simulink model "IF_with_EnabledSS"  (Simulink 9.0)
settings: Solver=FixedStepDiscrete  StartTime=0.0  StopTime=1  FixedStep=0.020000  MaxStep=1  RelTol=1e-3  EnableMultiTasking=on
model workspace (MAT data in the model file):
  x : num (value not decoded)
settings Model: SuppressorTable=22 serialization::archive 11 0 6 0 0 0 0 0  Creator=arnaud  LastModifiedBy=hbourbou
settings DataIOCC: LimitDataPoints=on  SaveFormat=Structure
settings DebuggingCC: UnderspecifiedInitializationDetection=Simplified  MergeDetectMultiDrivingBlocksExec=error  SolverPrmCheckMsg=warning
settings GRTTargetCC: GeneratePreprocessorConditionals=Disable all
settings ConfigComp: CovSFcnEnable=off

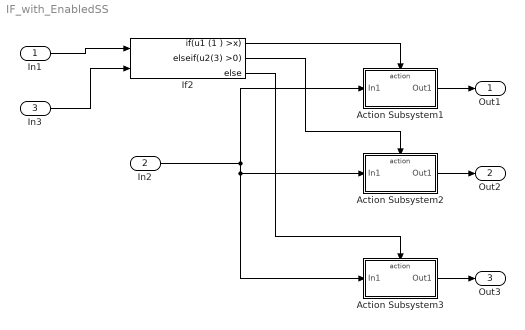
== system IF_with_EnabledSS ==
  In1 : Inport  PortDimensions=3
  In2 : Inport  Port=2
  In3 : Inport  Port=3  OutDataTypeStr=int32  PortDimensions=3
  Action Subsystem1 : Subsystem  TreatAsAtomicUnit=on
  Action Subsystem2 : Subsystem  TreatAsAtomicUnit=on
  Action Subsystem3 : Subsystem  TreatAsAtomicUnit=on
  If2 : If  NumInputs=2  IfExpression=u1 (1 ) >x  ElseIfExpressions=u2(3) >0
  Out1 : Outport
  Out2 : Outport  Port=2
  Out3 : Outport  Port=3
  wires:
  If2/1 -> Action Subsystem1/Action
  In1/1 -> If2/1
  If2/2 -> Action Subsystem2/Action
  Action Subsystem1/1(Out1) -> Out1/1
  Action Subsystem2/1(Out1) -> Out2/1
  In2/1 -> Action Subsystem3/1(In1), Action Subsystem2/1(In1), Action Subsystem1/1(In1)
  In3/1 -> If2/2
  If2/3 -> Action Subsystem3/Action
  Action Subsystem3/1(Out1) -> Out3/1

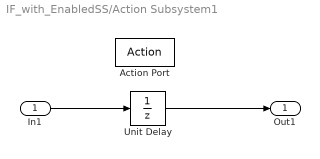
== system IF_with_EnabledSS/Action Subsystem1 ==
  In1 : Inport
  Action Port : ActionPort  InitializeStates=reset  ActionType=then
  Unit Delay : UnitDelay  SampleTime=-1
  Out1 : Outport
  wires:
  In1/1 -> Unit Delay/1
  Unit Delay/1 -> Out1/1

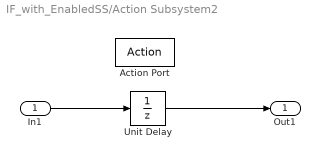
== system IF_with_EnabledSS/Action Subsystem2 ==
  In1 : Inport
  Action Port : ActionPort  ActionType=elseif
  Unit Delay : UnitDelay  SampleTime=-1
  Out1 : Outport
  wires:
  In1/1 -> Unit Delay/1
  Unit Delay/1 -> Out1/1

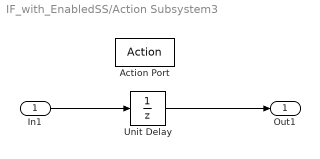
== system IF_with_EnabledSS/Action Subsystem3 ==
  In1 : Inport
  Action Port : ActionPort  ActionType=else
  Unit Delay : UnitDelay  SampleTime=-1
  Out1 : Outport
  wires:
  In1/1 -> Unit Delay/1
  Unit Delay/1 -> Out1/1
